simulink model "SdmTestbench"  (R2017a)
settings: Solver=VariableStepAuto  StartTime=0.0  StopTime=0.1  RelTol=1e-3
undefined symbols (not defined in the file): H, isLinearModel, isReferenceInput, sdm_q_sim, Ts
libraries: cstblocks x2
settings Model: Creator=bhannigan  LastModifiedBy=bhannigan

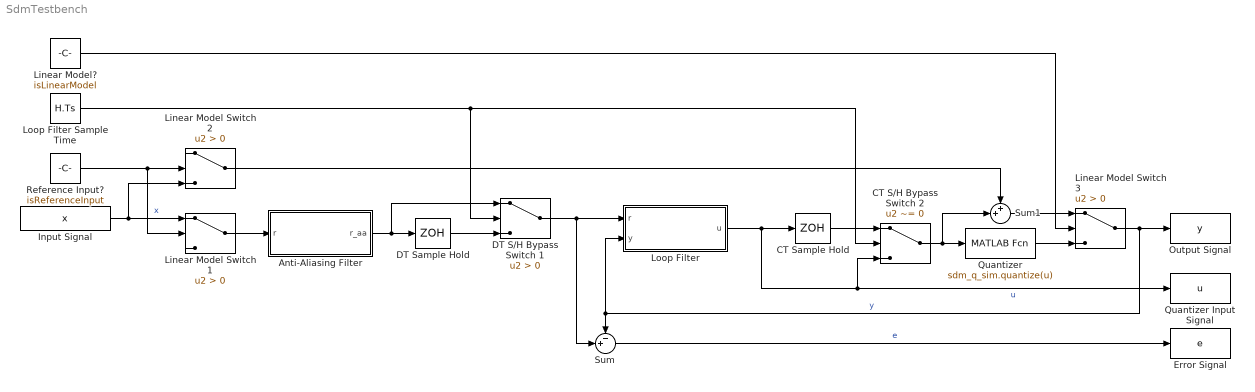
== system SdmTestbench ==
  Anti-Aliasing Filter : Subsystem
  CT S/H Bypass Switch 2 : Switch  Criteria=u2 ~= 0
  CT Sample Hold : ZeroOrderHold  SampleTime=Ts
  DT S/H Bypass Switch 1 : Switch  Criteria=u2 > Threshold
  DT Sample Hold : ZeroOrderHold  SampleTime=Ts
  Error Signal : ToWorkspace  VariableName=e  SaveFormat=Timeseries  SampleTime=-1
  Input Signal : FromWorkspace  VariableName=x  SampleTime=0
  Linear Model Switch 1 : Switch  Criteria=u2 > Threshold
  Linear Model Switch 2 : Switch  Criteria=u2 > Threshold
  Linear Model Switch 3 : Switch  Criteria=u2 > Threshold
  Linear Model? : Constant  Value=isLinearModel
  Loop Filter : Subsystem
  Loop Filter Sample Time : Constant  Value=H.Ts
  Output Signal : ToWorkspace  VariableName=y  SaveFormat=Timeseries  SampleTime=-1
  Quantizer : MATLABFcn  MATLABFcn=sdm_q_sim.quantize(u)
  Quantizer Input Signal : ToWorkspace  VariableName=u  SaveFormat=Timeseries  SampleTime=-1
  Reference Input? : Constant  Value=isReferenceInput
  Sum : Sum  Inputs=-+|
  Sum1 : Sum  Inputs=++|
  wires:
  Sum/1 -> Error Signal/1  "e"
  Loop Filter/1(u) -> CT Sample Hold/1, CT S/H Bypass Switch 2/3, Quantizer Input Signal/1  "u"
  Sum1/1 -> Linear Model Switch 3/1
  Linear Model?/1 -> Linear Model Switch 3/2
  Linear Model Switch 3/1 -> Output Signal/1, Sum/1, Loop Filter/2(y)  "y"
  CT Sample Hold/1 -> CT S/H Bypass Switch 2/1
  CT S/H Bypass Switch 2/1 -> Quantizer/1, Sum1/2
  Loop Filter Sample Time/1 -> DT S/H Bypass Switch 1/2, CT S/H Bypass Switch 2/2
  Anti-Aliasing Filter/1(r_aa) -> DT S/H Bypass Switch 1/1, DT Sample Hold/1
  DT Sample Hold/1 -> DT S/H Bypass Switch 1/3
  DT S/H Bypass Switch 1/1 -> Sum/2, Loop Filter/1(r)
  Linear Model Switch 1/1 -> Anti-Aliasing Filter/1(r)
  Linear Model Switch 2/1 -> Sum1/1
  Reference Input?/1 -> Linear Model Switch 1/2, Linear Model Switch 2/2
  Input Signal/1 -> Linear Model Switch 1/1, Linear Model Switch 2/3  "x"
  Quantizer/1 -> Linear Model Switch 3/3

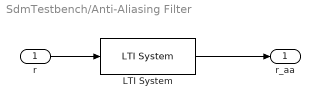
== system SdmTestbench/Anti-Aliasing Filter ==
  r : Inport
  LTI System : cstblocks/LTI System  sys=H_pre  IC=[]
  r_aa : Outport
  wires:
  r/1 -> LTI System/1
  LTI System/1 -> r_aa/1

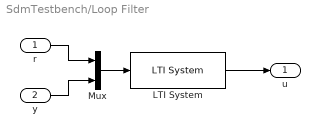
== system SdmTestbench/Loop Filter ==
  r : Inport
  y : Inport  Port=2
  LTI System : cstblocks/LTI System  sys=H  IC=[]
  Mux : Mux  Inputs=2
  u : Outport
  wires:
  r/1 -> Mux/1
  y/1 -> Mux/2
  Mux/1 -> LTI System/1
  LTI System/1 -> u/1
